simulink model "Project1_SPXMMA001"  (R2021a)
settings: Solver=ode1  StartTime=0.0  StopTime=Inf  RelTol=1e-3
InitFcn:
  |  TOFF_InitialValue.PRE = 12000;
  | OFF_InitialValue.PRE = 12000;
  | TON_InitialValue.PRE = 2000;
  | ON_InitialValue.PRE = 2000;
  | T2OFF_InitialValue.PRE = 11000;
  | T2ON_InitialValue.PRE = 3000;
  | T3OFF_InitialValue.PRE = 5000;
undefined symbols (not defined in the file): BOOL, DINT, slplc
libraries: simulink x7
(part 9 of 13)

== system Project1_SPXMMA001/PLC Controller Suite/__Logic/Task/Program/__Logic/TOF/Instruction_Enable/Initialize Function ==
  Constant : Constant  Value=0  OutDataTypeStr=BOOL
  Event Listener : EventListener  DisableCoverage=on  EventName=reset
  VarRead : Subsystem  DisableCoverage=on  TreatAsAtomicUnit=on  mask{PLCOperandTag=PRE, PLCOperandExpression=xxx_PLC_VAR_TOFF.PRE, PLCBlockType=VarRead, PLCPOUType=VarRead}
      mask prompts: PLCOperandTag "Operand Tag"
      mask init:
      | block = gcb;
      | maskObj = Simulink.Mask.get(block);
      | maskObj.Display = sprintf('disp(''%s'');', PLCOperandTag);
      | slplc.callbacks.initInstruction(gcb);
      mask Help: web([docroot '/plccoder/ref/varread' '.html']);
      mask DialogControl PLCBlockTitle Prompt: Variable Read
      mask Display: disp('PRE');
  VarWrite : Subsystem  DisableCoverage=on  TreatAsAtomicUnit=on  mask{PLCOperandTag=ACC, PLCOperandExpression=xxx_PLC_VAR_TOFF.ACC, PLCBlockType=VarWrite, PLCPOUType=VarWrite}
      mask prompts: PLCOperandTag "Operand Tag:"
      mask init:
      | slplc.callbacks.initInstruction(gcb);
      mask Help: web([docroot '/plccoder/ref/varwrite' '.html']);
      mask DialogControl PLCBlockTitle Prompt: Variable Write
      mask Display: disp(get_param(gcb, 'PLCOperandTag'));
  VarWrite1 : Subsystem  DisableCoverage=on  TreatAsAtomicUnit=on  mask{PLCOperandTag=EN, PLCOperandExpression=xxx_PLC_VAR_TOFF.EN, PLCBlockType=VarWrite, PLCPOUType=VarWrite}
      mask prompts: PLCOperandTag "Operand Tag:"
      mask init:
      | slplc.callbacks.initInstruction(gcb);
      mask Help: web([docroot '/plccoder/ref/varwrite' '.html']);
      mask DialogControl PLCBlockTitle Prompt: Variable Write
      mask Display: disp(get_param(gcb, 'PLCOperandTag'));
  VarWrite2 : Subsystem  DisableCoverage=on  TreatAsAtomicUnit=on  mask{PLCOperandTag=TT, PLCOperandExpression=xxx_PLC_VAR_TOFF.TT, PLCBlockType=VarWrite, PLCPOUType=VarWrite}
      mask prompts: PLCOperandTag "Operand Tag:"
      mask init:
      | slplc.callbacks.initInstruction(gcb);
      mask Help: web([docroot '/plccoder/ref/varwrite' '.html']);
      mask DialogControl PLCBlockTitle Prompt: Variable Write
      mask Display: disp(get_param(gcb, 'PLCOperandTag'));
  VarWrite3 : Subsystem  DisableCoverage=on  TreatAsAtomicUnit=on  mask{PLCOperandTag=DN, PLCOperandExpression=xxx_PLC_VAR_TOFF.DN, PLCBlockType=VarWrite, PLCPOUType=VarWrite}
      mask prompts: PLCOperandTag "Operand Tag:"
      mask init:
      | slplc.callbacks.initInstruction(gcb);
      mask Help: web([docroot '/plccoder/ref/varwrite' '.html']);
      mask DialogControl PLCBlockTitle Prompt: Variable Write
      mask Display: disp(get_param(gcb, 'PLCOperandTag'));
  wires:
  Constant/1 -> VarWrite1/1(In1), VarWrite2/1(In1), VarWrite3/1(In1)
  VarRead/1(Out1) -> VarWrite/1(In1)

== system Project1_SPXMMA001/PLC Controller Suite/__Logic/Task/Program/__Logic/TOF/Instruction_Enable/__CoreVarRead ==
  DataRead : DataStoreRead  DataStoreName=xxx_PLC_VAR_TOFF  IndexOptions=Index vector (dialog)  Indices=1  OutputSizes=1
  y : Outport  VectorParamsAs1DForOutWhenUnconnected=off
  wires:
  DataRead/1 -> y/1

== system Project1_SPXMMA001/PLC Controller Suite/__Logic/Task/Program/__Logic/TOF/Instruction_Enable/__CoreVarWrite ==
  u : Inport
  DataWrite : DataStoreWrite  DataStoreName=xxx_PLC_VAR_TOFF  IndexOptions=Index vector (dialog)  Indices=1  OutputSizes=1
  wires:
  u/1 -> DataWrite/1

== system Project1_SPXMMA001/PLC Controller Suite/__Logic/Task/Program/__Logic/TOF/RungInOverride/ForceRungInFalseRead ==
  __CoreLabelRead : Subsystem  Tag=CoreVarReadBlock  DisableCoverage=on  TreatAsAtomicUnit=on  mask{PLCBlockType=CoreLabelRead}
      mask init:
      | slplc.callbacks.initRoutineLabelRead(gcb);
      mask Help: web([docroot '/plccoder/ref/__corelabelread' '.html']);
      mask DialogControl PLCBlockTitle Prompt: Core Label Read
  Out1 : Outport  VectorParamsAs1DForOutWhenUnconnected=off
  wires:
  __CoreLabelRead/1(Out1) -> Out1/1

== system Project1_SPXMMA001/PLC Controller Suite/__Logic/Task/Program/__Logic/TOF1/BlockEnableRead/__CoreLabelRead ==
  DataRead : DataStoreRead  DataStoreName=x_PLCLabel__s4_3653__Block_Enable  IndexOptions=Index vector (dialog)  Indices=1  OutputSizes=1
  Out1 : Outport  VectorParamsAs1DForOutWhenUnconnected=off
  wires:
  DataRead/1 -> Out1/1

== system Project1_SPXMMA001/PLC Controller Suite/__Logic/Task/Program/__Logic/TOF1/Instruction_Enable/Initialize Function ==
  Constant : Constant  Value=0  OutDataTypeStr=BOOL
  Event Listener : EventListener  DisableCoverage=on  EventName=reset
  VarRead : Subsystem  DisableCoverage=on  TreatAsAtomicUnit=on  mask{PLCOperandTag=PRE, PLCOperandExpression=xxx_PLC_VAR_OFF.PRE, PLCBlockType=VarRead, PLCPOUType=VarRead}
      mask prompts: PLCOperandTag "Operand Tag"
      mask init:
      | block = gcb;
      | maskObj = Simulink.Mask.get(block);
      | maskObj.Display = sprintf('disp(''%s'');', PLCOperandTag);
      | slplc.callbacks.initInstruction(gcb);
      mask Help: web([docroot '/plccoder/ref/varread' '.html']);
      mask DialogControl PLCBlockTitle Prompt: Variable Read
      mask Display: disp('PRE');
  VarWrite : Subsystem  DisableCoverage=on  TreatAsAtomicUnit=on  mask{PLCOperandTag=ACC, PLCOperandExpression=xxx_PLC_VAR_OFF.ACC, PLCBlockType=VarWrite, PLCPOUType=VarWrite}
      mask prompts: PLCOperandTag "Operand Tag:"
      mask init:
      | slplc.callbacks.initInstruction(gcb);
      mask Help: web([docroot '/plccoder/ref/varwrite' '.html']);
      mask DialogControl PLCBlockTitle Prompt: Variable Write
      mask Display: disp(get_param(gcb, 'PLCOperandTag'));
  VarWrite1 : Subsystem  DisableCoverage=on  TreatAsAtomicUnit=on  mask{PLCOperandTag=EN, PLCOperandExpression=xxx_PLC_VAR_OFF.EN, PLCBlockType=VarWrite, PLCPOUType=VarWrite}
      mask prompts: PLCOperandTag "Operand Tag:"
      mask init:
      | slplc.callbacks.initInstruction(gcb);
      mask Help: web([docroot '/plccoder/ref/varwrite' '.html']);
      mask DialogControl PLCBlockTitle Prompt: Variable Write
      mask Display: disp(get_param(gcb, 'PLCOperandTag'));
  VarWrite2 : Subsystem  DisableCoverage=on  TreatAsAtomicUnit=on  mask{PLCOperandTag=TT, PLCOperandExpression=xxx_PLC_VAR_OFF.TT, PLCBlockType=VarWrite, PLCPOUType=VarWrite}
      mask prompts: PLCOperandTag "Operand Tag:"
      mask init:
      | slplc.callbacks.initInstruction(gcb);
      mask Help: web([docroot '/plccoder/ref/varwrite' '.html']);
      mask DialogControl PLCBlockTitle Prompt: Variable Write
      mask Display: disp(get_param(gcb, 'PLCOperandTag'));
  VarWrite3 : Subsystem  DisableCoverage=on  TreatAsAtomicUnit=on  mask{PLCOperandTag=DN, PLCOperandExpression=xxx_PLC_VAR_OFF.DN, PLCBlockType=VarWrite, PLCPOUType=VarWrite}
      mask prompts: PLCOperandTag "Operand Tag:"
      mask init:
      | slplc.callbacks.initInstruction(gcb);
      mask Help: web([docroot '/plccoder/ref/varwrite' '.html']);
      mask DialogControl PLCBlockTitle Prompt: Variable Write
      mask Display: disp(get_param(gcb, 'PLCOperandTag'));
  wires:
  Constant/1 -> VarWrite1/1(In1), VarWrite2/1(In1), VarWrite3/1(In1)
  VarRead/1(Out1) -> VarWrite/1(In1)

== system Project1_SPXMMA001/PLC Controller Suite/__Logic/Task/Program/__Logic/TOF1/Instruction_Enable/__CoreVarRead ==
  DataRead : DataStoreRead  DataStoreName=xxx_PLC_VAR_OFF  IndexOptions=Index vector (dialog)  Indices=1  OutputSizes=1
  y : Outport  VectorParamsAs1DForOutWhenUnconnected=off
  wires:
  DataRead/1 -> y/1

== system Project1_SPXMMA001/PLC Controller Suite/__Logic/Task/Program/__Logic/TOF1/Instruction_Enable/__CoreVarWrite ==
  u : Inport
  DataWrite : DataStoreWrite  DataStoreName=xxx_PLC_VAR_OFF  IndexOptions=Index vector (dialog)  Indices=1  OutputSizes=1
  wires:
  u/1 -> DataWrite/1

== system Project1_SPXMMA001/PLC Controller Suite/__Logic/Task/Program/__Logic/TOF1/RungInOverride/ForceRungInFalseRead ==
  __CoreLabelRead : Subsystem  Tag=CoreVarReadBlock  DisableCoverage=on  TreatAsAtomicUnit=on  mask{PLCBlockType=CoreLabelRead}
      mask init:
      | slplc.callbacks.initRoutineLabelRead(gcb);
      mask Help: web([docroot '/plccoder/ref/__corelabelread' '.html']);
      mask DialogControl PLCBlockTitle Prompt: Core Label Read
  Out1 : Outport  VectorParamsAs1DForOutWhenUnconnected=off
  wires:
  __CoreLabelRead/1(Out1) -> Out1/1

== system Project1_SPXMMA001/PLC Controller Suite/__Logic/Task/Program/__Logic/TOF2/BlockEnableRead/__CoreLabelRead ==
  DataRead : DataStoreRead  DataStoreName=x_PLCLabel__s4_3653__Block_Enable  IndexOptions=Index vector (dialog)  Indices=1  OutputSizes=1
  Out1 : Outport  VectorParamsAs1DForOutWhenUnconnected=off
  wires:
  DataRead/1 -> Out1/1

== system Project1_SPXMMA001/PLC Controller Suite/__Logic/Task/Program/__Logic/TOF2/Instruction_Enable/Initialize Function ==
  Constant : Constant  Value=0  OutDataTypeStr=BOOL
  Event Listener : EventListener  DisableCoverage=on  EventName=reset
  VarRead : Subsystem  DisableCoverage=on  TreatAsAtomicUnit=on  mask{PLCOperandTag=PRE, PLCOperandExpression=xxx_PLC_VAR_T2OFF.PRE, PLCBlockType=VarRead, PLCPOUType=VarRead}
      mask prompts: PLCOperandTag "Operand Tag"
      mask init:
      | block = gcb;
      | maskObj = Simulink.Mask.get(block);
      | maskObj.Display = sprintf('disp(''%s'');', PLCOperandTag);
      | slplc.callbacks.initInstruction(gcb);
      mask Help: web([docroot '/plccoder/ref/varread' '.html']);
      mask DialogControl PLCBlockTitle Prompt: Variable Read
      mask Display: disp('PRE');
  VarWrite : Subsystem  DisableCoverage=on  TreatAsAtomicUnit=on  mask{PLCOperandTag=ACC, PLCOperandExpression=xxx_PLC_VAR_T2OFF.ACC, PLCBlockType=VarWrite, PLCPOUType=VarWrite}
      mask prompts: PLCOperandTag "Operand Tag:"
      mask init:
      | slplc.callbacks.initInstruction(gcb);
      mask Help: web([docroot '/plccoder/ref/varwrite' '.html']);
      mask DialogControl PLCBlockTitle Prompt: Variable Write
      mask Display: disp(get_param(gcb, 'PLCOperandTag'));
  VarWrite1 : Subsystem  DisableCoverage=on  TreatAsAtomicUnit=on  mask{PLCOperandTag=EN, PLCOperandExpression=xxx_PLC_VAR_T2OFF.EN, PLCBlockType=VarWrite, PLCPOUType=VarWrite}
      mask prompts: PLCOperandTag "Operand Tag:"
      mask init:
      | slplc.callbacks.initInstruction(gcb);
      mask Help: web([docroot '/plccoder/ref/varwrite' '.html']);
      mask DialogControl PLCBlockTitle Prompt: Variable Write
      mask Display: disp(get_param(gcb, 'PLCOperandTag'));
  VarWrite2 : Subsystem  DisableCoverage=on  TreatAsAtomicUnit=on  mask{PLCOperandTag=TT, PLCOperandExpression=xxx_PLC_VAR_T2OFF.TT, PLCBlockType=VarWrite, PLCPOUType=VarWrite}
      mask prompts: PLCOperandTag "Operand Tag:"
      mask init:
      | slplc.callbacks.initInstruction(gcb);
      mask Help: web([docroot '/plccoder/ref/varwrite' '.html']);
      mask DialogControl PLCBlockTitle Prompt: Variable Write
      mask Display: disp(get_param(gcb, 'PLCOperandTag'));
  VarWrite3 : Subsystem  DisableCoverage=on  TreatAsAtomicUnit=on  mask{PLCOperandTag=DN, PLCOperandExpression=xxx_PLC_VAR_T2OFF.DN, PLCBlockType=VarWrite, PLCPOUType=VarWrite}
      mask prompts: PLCOperandTag "Operand Tag:"
      mask init:
      | slplc.callbacks.initInstruction(gcb);
      mask Help: web([docroot '/plccoder/ref/varwrite' '.html']);
      mask DialogControl PLCBlockTitle Prompt: Variable Write
      mask Display: disp(get_param(gcb, 'PLCOperandTag'));
  wires:
  Constant/1 -> VarWrite1/1(In1), VarWrite2/1(In1), VarWrite3/1(In1)
  VarRead/1(Out1) -> VarWrite/1(In1)

== system Project1_SPXMMA001/PLC Controller Suite/__Logic/Task/Program/__Logic/TOF2/Instruction_Enable/__CoreVarRead ==
  DataRead : DataStoreRead  DataStoreName=xxx_PLC_VAR_T2OFF  IndexOptions=Index vector (dialog)  Indices=1  OutputSizes=1
  y : Outport  VectorParamsAs1DForOutWhenUnconnected=off
  wires:
  DataRead/1 -> y/1

== system Project1_SPXMMA001/PLC Controller Suite/__Logic/Task/Program/__Logic/TOF2/Instruction_Enable/__CoreVarWrite ==
  u : Inport
  DataWrite : DataStoreWrite  DataStoreName=xxx_PLC_VAR_T2OFF  IndexOptions=Index vector (dialog)  Indices=1  OutputSizes=1
  wires:
  u/1 -> DataWrite/1

== system Project1_SPXMMA001/PLC Controller Suite/__Logic/Task/Program/__Logic/TOF2/RungInOverride/ForceRungInFalseRead ==
  __CoreLabelRead : Subsystem  Tag=CoreVarReadBlock  DisableCoverage=on  TreatAsAtomicUnit=on  mask{PLCBlockType=CoreLabelRead}
      mask init:
      | slplc.callbacks.initRoutineLabelRead(gcb);
      mask Help: web([docroot '/plccoder/ref/__corelabelread' '.html']);
      mask DialogControl PLCBlockTitle Prompt: Core Label Read
  Out1 : Outport  VectorParamsAs1DForOutWhenUnconnected=off
  wires:
  __CoreLabelRead/1(Out1) -> Out1/1

== system Project1_SPXMMA001/PLC Controller Suite/__Logic/Task/Program/__Logic/TOF3/BlockEnableRead/__CoreLabelRead ==
  DataRead : DataStoreRead  DataStoreName=x_PLCLabel__s4_3653__Block_Enable  IndexOptions=Index vector (dialog)  Indices=1  OutputSizes=1
  Out1 : Outport  VectorParamsAs1DForOutWhenUnconnected=off
  wires:
  DataRead/1 -> Out1/1

== system Project1_SPXMMA001/PLC Controller Suite/__Logic/Task/Program/__Logic/TOF3/Instruction_Enable/Initialize Function ==
  Constant : Constant  Value=0  OutDataTypeStr=BOOL
  Event Listener : EventListener  DisableCoverage=on  EventName=reset
  VarRead : Subsystem  DisableCoverage=on  TreatAsAtomicUnit=on  mask{PLCOperandTag=PRE, PLCOperandExpression=xxx_PLC_VAR_T3OFF.PRE, PLCBlockType=VarRead, PLCPOUType=VarRead}
      mask prompts: PLCOperandTag "Operand Tag"
      mask init:
      | block = gcb;
      | maskObj = Simulink.Mask.get(block);
      | maskObj.Display = sprintf('disp(''%s'');', PLCOperandTag);
      | slplc.callbacks.initInstruction(gcb);
      mask Help: web([docroot '/plccoder/ref/varread' '.html']);
      mask DialogControl PLCBlockTitle Prompt: Variable Read
      mask Display: disp('PRE');
  VarWrite : Subsystem  DisableCoverage=on  TreatAsAtomicUnit=on  mask{PLCOperandTag=ACC, PLCOperandExpression=xxx_PLC_VAR_T3OFF.ACC, PLCBlockType=VarWrite, PLCPOUType=VarWrite}
      mask prompts: PLCOperandTag "Operand Tag:"
      mask init:
      | slplc.callbacks.initInstruction(gcb);
      mask Help: web([docroot '/plccoder/ref/varwrite' '.html']);
      mask DialogControl PLCBlockTitle Prompt: Variable Write
      mask Display: disp(get_param(gcb, 'PLCOperandTag'));
  VarWrite1 : Subsystem  DisableCoverage=on  TreatAsAtomicUnit=on  mask{PLCOperandTag=EN, PLCOperandExpression=xxx_PLC_VAR_T3OFF.EN, PLCBlockType=VarWrite, PLCPOUType=VarWrite}
      mask prompts: PLCOperandTag "Operand Tag:"
      mask init:
      | slplc.callbacks.initInstruction(gcb);
      mask Help: web([docroot '/plccoder/ref/varwrite' '.html']);
      mask DialogControl PLCBlockTitle Prompt: Variable Write
      mask Display: disp(get_param(gcb, 'PLCOperandTag'));
  VarWrite2 : Subsystem  DisableCoverage=on  TreatAsAtomicUnit=on  mask{PLCOperandTag=TT, PLCOperandExpression=xxx_PLC_VAR_T3OFF.TT, PLCBlockType=VarWrite, PLCPOUType=VarWrite}
      mask prompts: PLCOperandTag "Operand Tag:"
      mask init:
      | slplc.callbacks.initInstruction(gcb);
      mask Help: web([docroot '/plccoder/ref/varwrite' '.html']);
      mask DialogControl PLCBlockTitle Prompt: Variable Write
      mask Display: disp(get_param(gcb, 'PLCOperandTag'));
  VarWrite3 : Subsystem  DisableCoverage=on  TreatAsAtomicUnit=on  mask{PLCOperandTag=DN, PLCOperandExpression=xxx_PLC_VAR_T3OFF.DN, PLCBlockType=VarWrite, PLCPOUType=VarWrite}
      mask prompts: PLCOperandTag "Operand Tag:"
      mask init:
      | slplc.callbacks.initInstruction(gcb);
      mask Help: web([docroot '/plccoder/ref/varwrite' '.html']);
      mask DialogControl PLCBlockTitle Prompt: Variable Write
      mask Display: disp(get_param(gcb, 'PLCOperandTag'));
  wires:
  Constant/1 -> VarWrite1/1(In1), VarWrite2/1(In1), VarWrite3/1(In1)
  VarRead/1(Out1) -> VarWrite/1(In1)

== system Project1_SPXMMA001/PLC Controller Suite/__Logic/Task/Program/__Logic/TOF3/Instruction_Enable/__CoreVarRead ==
  DataRead : DataStoreRead  DataStoreName=xxx_PLC_VAR_T3OFF  IndexOptions=Index vector (dialog)  Indices=1  OutputSizes=1
  y : Outport  VectorParamsAs1DForOutWhenUnconnected=off
  wires:
  DataRead/1 -> y/1

== system Project1_SPXMMA001/PLC Controller Suite/__Logic/Task/Program/__Logic/TOF3/Instruction_Enable/__CoreVarWrite ==
  u : Inport
  DataWrite : DataStoreWrite  DataStoreName=xxx_PLC_VAR_T3OFF  IndexOptions=Index vector (dialog)  Indices=1  OutputSizes=1
  wires:
  u/1 -> DataWrite/1

== system Project1_SPXMMA001/PLC Controller Suite/__Logic/Task/Program/__Logic/TOF3/RungInOverride/ForceRungInFalseRead ==
  __CoreLabelRead : Subsystem  Tag=CoreVarReadBlock  DisableCoverage=on  TreatAsAtomicUnit=on  mask{PLCBlockType=CoreLabelRead}
      mask init:
      | slplc.callbacks.initRoutineLabelRead(gcb);
      mask Help: web([docroot '/plccoder/ref/__corelabelread' '.html']);
      mask DialogControl PLCBlockTitle Prompt: Core Label Read
  Out1 : Outport  VectorParamsAs1DForOutWhenUnconnected=off
  wires:
  __CoreLabelRead/1(Out1) -> Out1/1

== system Project1_SPXMMA001/PLC Controller Suite/__Logic/Task/Program/__Logic/TON/BlockEnableRead/__CoreLabelRead ==
  DataRead : DataStoreRead  DataStoreName=x_PLCLabel__s4_3653__Block_Enable  IndexOptions=Index vector (dialog)  Indices=1  OutputSizes=1
  Out1 : Outport  VectorParamsAs1DForOutWhenUnconnected=off
  wires:
  DataRead/1 -> Out1/1

== system Project1_SPXMMA001/PLC Controller Suite/__Logic/Task/Program/__Logic/TON/Instruction_Enable/Initialize Function ==
  Constant : Constant  Value=0  OutDataTypeStr=BOOL
  Constant1 : Constant  Value=0  OutDataTypeStr=DINT
  Event Listener : EventListener  DisableCoverage=on  EventName=reset
  VarWrite : Subsystem  DisableCoverage=on  TreatAsAtomicUnit=on  mask{PLCOperandTag=ACC, PLCOperandExpression=xxx_PLC_VAR_TON.ACC, PLCBlockType=VarWrite, PLCPOUType=VarWrite}
      mask prompts: PLCOperandTag "Operand Tag:"
      mask init:
      | slplc.callbacks.initInstruction(gcb);
      mask Help: web([docroot '/plccoder/ref/varwrite' '.html']);
      mask DialogControl PLCBlockTitle Prompt: Variable Write
      mask Display: disp(get_param(gcb, 'PLCOperandTag'));
  VarWrite1 : Subsystem  DisableCoverage=on  TreatAsAtomicUnit=on  mask{PLCOperandTag=EN, PLCOperandExpression=xxx_PLC_VAR_TON.EN, PLCBlockType=VarWrite, PLCPOUType=VarWrite}
      mask prompts: PLCOperandTag "Operand Tag:"
      mask init:
      | slplc.callbacks.initInstruction(gcb);
      mask Help: web([docroot '/plccoder/ref/varwrite' '.html']);
      mask DialogControl PLCBlockTitle Prompt: Variable Write
      mask Display: disp(get_param(gcb, 'PLCOperandTag'));
  VarWrite2 : Subsystem  DisableCoverage=on  TreatAsAtomicUnit=on  mask{PLCOperandTag=TT, PLCOperandExpression=xxx_PLC_VAR_TON.TT, PLCBlockType=VarWrite, PLCPOUType=VarWrite}
      mask prompts: PLCOperandTag "Operand Tag:"
      mask init:
      | slplc.callbacks.initInstruction(gcb);
      mask Help: web([docroot '/plccoder/ref/varwrite' '.html']);
      mask DialogControl PLCBlockTitle Prompt: Variable Write
      mask Display: disp(get_param(gcb, 'PLCOperandTag'));
  VarWrite3 : Subsystem  DisableCoverage=on  TreatAsAtomicUnit=on  mask{PLCOperandTag=DN, PLCOperandExpression=xxx_PLC_VAR_TON.DN, PLCBlockType=VarWrite, PLCPOUType=VarWrite}
      mask prompts: PLCOperandTag "Operand Tag:"
      mask init:
      | slplc.callbacks.initInstruction(gcb);
      mask Help: web([docroot '/plccoder/ref/varwrite' '.html']);
      mask DialogControl PLCBlockTitle Prompt: Variable Write
      mask Display: disp(get_param(gcb, 'PLCOperandTag'));
  wires:
  Constant/1 -> VarWrite1/1(In1), VarWrite2/1(In1), VarWrite3/1(In1)
  Constant1/1 -> VarWrite/1(In1)

== system Project1_SPXMMA001/PLC Controller Suite/__Logic/Task/Program/__Logic/TON/Instruction_Enable/__CoreVarRead ==
  DataRead : DataStoreRead  DataStoreName=xxx_PLC_VAR_TON  IndexOptions=Index vector (dialog)  Indices=1  OutputSizes=1
  y : Outport  VectorParamsAs1DForOutWhenUnconnected=off
  wires:
  DataRead/1 -> y/1

== system Project1_SPXMMA001/PLC Controller Suite/__Logic/Task/Program/__Logic/TON/Instruction_Enable/__CoreVarWrite ==
  u : Inport
  DataWrite : DataStoreWrite  DataStoreName=xxx_PLC_VAR_TON  IndexOptions=Index vector (dialog)  Indices=1  OutputSizes=1
  wires:
  u/1 -> DataWrite/1

== system Project1_SPXMMA001/PLC Controller Suite/__Logic/Task/Program/__Logic/TON/RungInOverride/ForceRungInFalseRead ==
  __CoreLabelRead : Subsystem  Tag=CoreVarReadBlock  DisableCoverage=on  TreatAsAtomicUnit=on  mask{PLCBlockType=CoreLabelRead}
      mask init:
      | slplc.callbacks.initRoutineLabelRead(gcb);
      mask Help: web([docroot '/plccoder/ref/__corelabelread' '.html']);
      mask DialogControl PLCBlockTitle Prompt: Core Label Read
  Out1 : Outport  VectorParamsAs1DForOutWhenUnconnected=off
  wires:
  __CoreLabelRead/1(Out1) -> Out1/1

== system Project1_SPXMMA001/PLC Controller Suite/__Logic/Task/Program/__Logic/TON1/BlockEnableRead/__CoreLabelRead ==
  DataRead : DataStoreRead  DataStoreName=x_PLCLabel__s4_3653__Block_Enable  IndexOptions=Index vector (dialog)  Indices=1  OutputSizes=1
  Out1 : Outport  VectorParamsAs1DForOutWhenUnconnected=off
  wires:
  DataRead/1 -> Out1/1

== system Project1_SPXMMA001/PLC Controller Suite/__Logic/Task/Program/__Logic/TON1/Instruction_Enable/Initialize Function ==
  Constant : Constant  Value=0  OutDataTypeStr=BOOL
  Constant1 : Constant  Value=0  OutDataTypeStr=DINT
  Event Listener : EventListener  DisableCoverage=on  EventName=reset
  VarWrite : Subsystem  DisableCoverage=on  TreatAsAtomicUnit=on  mask{PLCOperandTag=ACC, PLCOperandExpression=xxx_PLC_VAR_ON.ACC, PLCBlockType=VarWrite, PLCPOUType=VarWrite}
      mask prompts: PLCOperandTag "Operand Tag:"
      mask init:
      | slplc.callbacks.initInstruction(gcb);
      mask Help: web([docroot '/plccoder/ref/varwrite' '.html']);
      mask DialogControl PLCBlockTitle Prompt: Variable Write
      mask Display: disp(get_param(gcb, 'PLCOperandTag'));
  VarWrite1 : Subsystem  DisableCoverage=on  TreatAsAtomicUnit=on  mask{PLCOperandTag=EN, PLCOperandExpression=xxx_PLC_VAR_ON.EN, PLCBlockType=VarWrite, PLCPOUType=VarWrite}
      mask prompts: PLCOperandTag "Operand Tag:"
      mask init:
      | slplc.callbacks.initInstruction(gcb);
      mask Help: web([docroot '/plccoder/ref/varwrite' '.html']);
      mask DialogControl PLCBlockTitle Prompt: Variable Write
      mask Display: disp(get_param(gcb, 'PLCOperandTag'));
  VarWrite2 : Subsystem  DisableCoverage=on  TreatAsAtomicUnit=on  mask{PLCOperandTag=TT, PLCOperandExpression=xxx_PLC_VAR_ON.TT, PLCBlockType=VarWrite, PLCPOUType=VarWrite}
      mask prompts: PLCOperandTag "Operand Tag:"
      mask init:
      | slplc.callbacks.initInstruction(gcb);
      mask Help: web([docroot '/plccoder/ref/varwrite' '.html']);
      mask DialogControl PLCBlockTitle Prompt: Variable Write
      mask Display: disp(get_param(gcb, 'PLCOperandTag'));
  VarWrite3 : Subsystem  DisableCoverage=on  TreatAsAtomicUnit=on  mask{PLCOperandTag=DN, PLCOperandExpression=xxx_PLC_VAR_ON.DN, PLCBlockType=VarWrite, PLCPOUType=VarWrite}
      mask prompts: PLCOperandTag "Operand Tag:"
      mask init:
      | slplc.callbacks.initInstruction(gcb);
      mask Help: web([docroot '/plccoder/ref/varwrite' '.html']);
      mask DialogControl PLCBlockTitle Prompt: Variable Write
      mask Display: disp(get_param(gcb, 'PLCOperandTag'));
  wires:
  Constant/1 -> VarWrite1/1(In1), VarWrite2/1(In1), VarWrite3/1(In1)
  Constant1/1 -> VarWrite/1(In1)

== system Project1_SPXMMA001/PLC Controller Suite/__Logic/Task/Program/__Logic/TON1/Instruction_Enable/__CoreVarRead ==
  DataRead : DataStoreRead  DataStoreName=xxx_PLC_VAR_ON  IndexOptions=Index vector (dialog)  Indices=1  OutputSizes=1
  y : Outport  VectorParamsAs1DForOutWhenUnconnected=off
  wires:
  DataRead/1 -> y/1

== system Project1_SPXMMA001/PLC Controller Suite/__Logic/Task/Program/__Logic/TON1/Instruction_Enable/__CoreVarWrite ==
  u : Inport
  DataWrite : DataStoreWrite  DataStoreName=xxx_PLC_VAR_ON  IndexOptions=Index vector (dialog)  Indices=1  OutputSizes=1
  wires:
  u/1 -> DataWrite/1

== system Project1_SPXMMA001/PLC Controller Suite/__Logic/Task/Program/__Logic/TON1/RungInOverride/ForceRungInFalseRead ==
  __CoreLabelRead : Subsystem  Tag=CoreVarReadBlock  DisableCoverage=on  TreatAsAtomicUnit=on  mask{PLCBlockType=CoreLabelRead}
      mask init:
      | slplc.callbacks.initRoutineLabelRead(gcb);
      mask Help: web([docroot '/plccoder/ref/__corelabelread' '.html']);
      mask DialogControl PLCBlockTitle Prompt: Core Label Read
  Out1 : Outport  VectorParamsAs1DForOutWhenUnconnected=off
  wires:
  __CoreLabelRead/1(Out1) -> Out1/1

== system Project1_SPXMMA001/PLC Controller Suite/__Logic/Task/Program/__Logic/TON2/BlockEnableRead/__CoreLabelRead ==
  DataRead : DataStoreRead  DataStoreName=x_PLCLabel__s4_3653__Block_Enable  IndexOptions=Index vector (dialog)  Indices=1  OutputSizes=1
  Out1 : Outport  VectorParamsAs1DForOutWhenUnconnected=off
  wires:
  DataRead/1 -> Out1/1

== system Project1_SPXMMA001/PLC Controller Suite/__Logic/Task/Program/__Logic/TON2/Instruction_Enable/Initialize Function ==
  Constant : Constant  Value=0  OutDataTypeStr=BOOL
  Constant1 : Constant  Value=0  OutDataTypeStr=DINT
  Event Listener : EventListener  DisableCoverage=on  EventName=reset
  VarWrite : Subsystem  DisableCoverage=on  TreatAsAtomicUnit=on  mask{PLCOperandTag=ACC, PLCOperandExpression=xxx_PLC_VAR_T2ON.ACC, PLCBlockType=VarWrite, PLCPOUType=VarWrite}
      mask prompts: PLCOperandTag "Operand Tag:"
      mask init:
      | slplc.callbacks.initInstruction(gcb);
      mask Help: web([docroot '/plccoder/ref/varwrite' '.html']);
      mask DialogControl PLCBlockTitle Prompt: Variable Write
      mask Display: disp(get_param(gcb, 'PLCOperandTag'));
  VarWrite1 : Subsystem  DisableCoverage=on  TreatAsAtomicUnit=on  mask{PLCOperandTag=EN, PLCOperandExpression=xxx_PLC_VAR_T2ON.EN, PLCBlockType=VarWrite, PLCPOUType=VarWrite}
      mask prompts: PLCOperandTag "Operand Tag:"
      mask init:
      | slplc.callbacks.initInstruction(gcb);
      mask Help: web([docroot '/plccoder/ref/varwrite' '.html']);
      mask DialogControl PLCBlockTitle Prompt: Variable Write
      mask Display: disp(get_param(gcb, 'PLCOperandTag'));
  VarWrite2 : Subsystem  DisableCoverage=on  TreatAsAtomicUnit=on  mask{PLCOperandTag=TT, PLCOperandExpression=xxx_PLC_VAR_T2ON.TT, PLCBlockType=VarWrite, PLCPOUType=VarWrite}
      mask prompts: PLCOperandTag "Operand Tag:"
      mask init:
      | slplc.callbacks.initInstruction(gcb);
      mask Help: web([docroot '/plccoder/ref/varwrite' '.html']);
      mask DialogControl PLCBlockTitle Prompt: Variable Write
      mask Display: disp(get_param(gcb, 'PLCOperandTag'));
  VarWrite3 : Subsystem  DisableCoverage=on  TreatAsAtomicUnit=on  mask{PLCOperandTag=DN, PLCOperandExpression=xxx_PLC_VAR_T2ON.DN, PLCBlockType=VarWrite, PLCPOUType=VarWrite}
      mask prompts: PLCOperandTag "Operand Tag:"
      mask init:
      | slplc.callbacks.initInstruction(gcb);
      mask Help: web([docroot '/plccoder/ref/varwrite' '.html']);
      mask DialogControl PLCBlockTitle Prompt: Variable Write
      mask Display: disp(get_param(gcb, 'PLCOperandTag'));
  wires:
  Constant/1 -> VarWrite1/1(In1), VarWrite2/1(In1), VarWrite3/1(In1)
  Constant1/1 -> VarWrite/1(In1)

== system Project1_SPXMMA001/PLC Controller Suite/__Logic/Task/Program/__Logic/TON2/Instruction_Enable/__CoreVarRead ==
  DataRead : DataStoreRead  DataStoreName=xxx_PLC_VAR_T2ON  IndexOptions=Index vector (dialog)  Indices=1  OutputSizes=1
  y : Outport  VectorParamsAs1DForOutWhenUnconnected=off
  wires:
  DataRead/1 -> y/1

== system Project1_SPXMMA001/PLC Controller Suite/__Logic/Task/Program/__Logic/TON2/Instruction_Enable/__CoreVarWrite ==
  u : Inport
  DataWrite : DataStoreWrite  DataStoreName=xxx_PLC_VAR_T2ON  IndexOptions=Index vector (dialog)  Indices=1  OutputSizes=1
  wires:
  u/1 -> DataWrite/1

== system Project1_SPXMMA001/PLC Controller Suite/__Logic/Task/Program/__Logic/TON2/RungInOverride/ForceRungInFalseRead ==
  __CoreLabelRead : Subsystem  Tag=CoreVarReadBlock  DisableCoverage=on  TreatAsAtomicUnit=on  mask{PLCBlockType=CoreLabelRead}
      mask init:
      | slplc.callbacks.initRoutineLabelRead(gcb);
      mask Help: web([docroot '/plccoder/ref/__corelabelread' '.html']);
      mask DialogControl PLCBlockTitle Prompt: Core Label Read
  Out1 : Outport  VectorParamsAs1DForOutWhenUnconnected=off
  wires:
  __CoreLabelRead/1(Out1) -> Out1/1

== system Project1_SPXMMA001/PLC Controller Suite/__Logic/Task/Program/__Logic/XIC/BlockEnableRead/__CoreLabelRead ==
  DataRead : DataStoreRead  DataStoreName=x_PLCLabel__s4_3653__Block_Enable  IndexOptions=Index vector (dialog)  Indices=1  OutputSizes=1
  Out1 : Outport  VectorParamsAs1DForOutWhenUnconnected=off
  wires:
  DataRead/1 -> Out1/1

== system Project1_SPXMMA001/PLC Controller Suite/__Logic/Task/Program/__Logic/XIC/Instruction_Enable/__CoreVarRead ==
  DataRead : DataStoreRead  DataStoreName=xxx_PLC_VAR_PED1_1  IndexOptions=Index vector (dialog)  Indices=1  OutputSizes=1
  y : Outport  VectorParamsAs1DForOutWhenUnconnected=off
  wires:
  DataRead/1 -> y/1

== system Project1_SPXMMA001/PLC Controller Suite/__Logic/Task/Program/__Logic/XIC/RungInOverride/ForceRungInFalseRead ==
  __CoreLabelRead : Subsystem  Tag=CoreVarReadBlock  DisableCoverage=on  TreatAsAtomicUnit=on  mask{PLCBlockType=CoreLabelRead}
      mask init:
      | slplc.callbacks.initRoutineLabelRead(gcb);
      mask Help: web([docroot '/plccoder/ref/__corelabelread' '.html']);
      mask DialogControl PLCBlockTitle Prompt: Core Label Read
  Out1 : Outport  VectorParamsAs1DForOutWhenUnconnected=off
  wires:
  __CoreLabelRead/1(Out1) -> Out1/1

== system Project1_SPXMMA001/PLC Controller Suite/__Logic/Task/Program/__Logic/XIC1/BlockEnableRead/__CoreLabelRead ==
  DataRead : DataStoreRead  DataStoreName=x_PLCLabel__s4_3653__Block_Enable  IndexOptions=Index vector (dialog)  Indices=1  OutputSizes=1
  Out1 : Outport  VectorParamsAs1DForOutWhenUnconnected=off
  wires:
  DataRead/1 -> Out1/1

== system Project1_SPXMMA001/PLC Controller Suite/__Logic/Task/Program/__Logic/XIC1/Instruction_Enable/__CoreVarRead ==
  DataRead : DataStoreRead  DataStoreName=xxx_PLC_VAR_PED1_2  IndexOptions=Index vector (dialog)  Indices=1  OutputSizes=1
  y : Outport  VectorParamsAs1DForOutWhenUnconnected=off
  wires:
  DataRead/1 -> y/1

== system Project1_SPXMMA001/PLC Controller Suite/__Logic/Task/Program/__Logic/XIC1/RungInOverride/ForceRungInFalseRead ==
  __CoreLabelRead : Subsystem  Tag=CoreVarReadBlock  DisableCoverage=on  TreatAsAtomicUnit=on  mask{PLCBlockType=CoreLabelRead}
      mask init:
      | slplc.callbacks.initRoutineLabelRead(gcb);
      mask Help: web([docroot '/plccoder/ref/__corelabelread' '.html']);
      mask DialogControl PLCBlockTitle Prompt: Core Label Read
  Out1 : Outport  VectorParamsAs1DForOutWhenUnconnected=off
  wires:
  __CoreLabelRead/1(Out1) -> Out1/1

== system Project1_SPXMMA001/PLC Controller Suite/__Logic/Task/Program/__Logic/XIC10/BlockEnableRead/__CoreLabelRead ==
  DataRead : DataStoreRead  DataStoreName=x_PLCLabel__s4_3653__Block_Enable  IndexOptions=Index vector (dialog)  Indices=1  OutputSizes=1
  Out1 : Outport  VectorParamsAs1DForOutWhenUnconnected=off
  wires:
  DataRead/1 -> Out1/1

== system Project1_SPXMMA001/PLC Controller Suite/__Logic/Task/Program/__Logic/XIC10/Instruction_Enable/__CoreVarRead ==
  DataRead : DataStoreRead  DataStoreName=xxx_PLC_VAR_T2ON  DataStoreElements=xxx_PLC_VAR_T2ON.DN  IndexOptions=Index vector (dialog)  Indices=1  OutputSizes=1
  y : Outport  VectorParamsAs1DForOutWhenUnconnected=off
  wires:
  DataRead/1 -> y/1

== system Project1_SPXMMA001/PLC Controller Suite/__Logic/Task/Program/__Logic/XIC10/RungInOverride/ForceRungInFalseRead ==
  __CoreLabelRead : Subsystem  Tag=CoreVarReadBlock  DisableCoverage=on  TreatAsAtomicUnit=on  mask{PLCBlockType=CoreLabelRead}
      mask init:
      | slplc.callbacks.initRoutineLabelRead(gcb);
      mask Help: web([docroot '/plccoder/ref/__corelabelread' '.html']);
      mask DialogControl PLCBlockTitle Prompt: Core Label Read
  Out1 : Outport  VectorParamsAs1DForOutWhenUnconnected=off
  wires:
  __CoreLabelRead/1(Out1) -> Out1/1

== system Project1_SPXMMA001/PLC Controller Suite/__Logic/Task/Program/__Logic/XIC11/BlockEnableRead/__CoreLabelRead ==
  DataRead : DataStoreRead  DataStoreName=x_PLCLabel__s4_3653__Block_Enable  IndexOptions=Index vector (dialog)  Indices=1  OutputSizes=1
  Out1 : Outport  VectorParamsAs1DForOutWhenUnconnected=off
  wires:
  DataRead/1 -> Out1/1

== system Project1_SPXMMA001/PLC Controller Suite/__Logic/Task/Program/__Logic/XIC11/Instruction_Enable/__CoreVarRead ==
  DataRead : DataStoreRead  DataStoreName=xxx_PLC_VAR_ZONE1_SENSOR  IndexOptions=Index vector (dialog)  Indices=1  OutputSizes=1
  y : Outport  VectorParamsAs1DForOutWhenUnconnected=off
  wires:
  DataRead/1 -> y/1

== system Project1_SPXMMA001/PLC Controller Suite/__Logic/Task/Program/__Logic/XIC11/RungInOverride/ForceRungInFalseRead ==
  __CoreLabelRead : Subsystem  Tag=CoreVarReadBlock  DisableCoverage=on  TreatAsAtomicUnit=on  mask{PLCBlockType=CoreLabelRead}
      mask init:
      | slplc.callbacks.initRoutineLabelRead(gcb);
      mask Help: web([docroot '/plccoder/ref/__corelabelread' '.html']);
      mask DialogControl PLCBlockTitle Prompt: Core Label Read
  Out1 : Outport  VectorParamsAs1DForOutWhenUnconnected=off
  wires:
  __CoreLabelRead/1(Out1) -> Out1/1

== system Project1_SPXMMA001/PLC Controller Suite/__Logic/Task/Program/__Logic/XIC12/BlockEnableRead/__CoreLabelRead ==
  DataRead : DataStoreRead  DataStoreName=x_PLCLabel__s4_3653__Block_Enable  IndexOptions=Index vector (dialog)  Indices=1  OutputSizes=1
  Out1 : Outport  VectorParamsAs1DForOutWhenUnconnected=off
  wires:
  DataRead/1 -> Out1/1

== system Project1_SPXMMA001/PLC Controller Suite/__Logic/Task/Program/__Logic/XIC12/Instruction_Enable/__CoreVarRead ==
  DataRead : DataStoreRead  DataStoreName=xxx_PLC_VAR_ZONE1_SENSOR  IndexOptions=Index vector (dialog)  Indices=1  OutputSizes=1
  y : Outport  VectorParamsAs1DForOutWhenUnconnected=off
  wires:
  DataRead/1 -> y/1

== system Project1_SPXMMA001/PLC Controller Suite/__Logic/Task/Program/__Logic/XIC12/RungInOverride/ForceRungInFalseRead ==
  __CoreLabelRead : Subsystem  Tag=CoreVarReadBlock  DisableCoverage=on  TreatAsAtomicUnit=on  mask{PLCBlockType=CoreLabelRead}
      mask init:
      | slplc.callbacks.initRoutineLabelRead(gcb);
      mask Help: web([docroot '/plccoder/ref/__corelabelread' '.html']);
      mask DialogControl PLCBlockTitle Prompt: Core Label Read
  Out1 : Outport  VectorParamsAs1DForOutWhenUnconnected=off
  wires:
  __CoreLabelRead/1(Out1) -> Out1/1

== system Project1_SPXMMA001/PLC Controller Suite/__Logic/Task/Program/__Logic/XIC13/BlockEnableRead/__CoreLabelRead ==
  DataRead : DataStoreRead  DataStoreName=x_PLCLabel__s4_3653__Block_Enable  IndexOptions=Index vector (dialog)  Indices=1  OutputSizes=1
  Out1 : Outport  VectorParamsAs1DForOutWhenUnconnected=off
  wires:
  DataRead/1 -> Out1/1

== system Project1_SPXMMA001/PLC Controller Suite/__Logic/Task/Program/__Logic/XIC13/Instruction_Enable/__CoreVarRead ==
  DataRead : DataStoreRead  DataStoreName=xxx_PLC_VAR_ZONE2  IndexOptions=Index vector (dialog)  Indices=1  OutputSizes=1
  y : Outport  VectorParamsAs1DForOutWhenUnconnected=off
  wires:
  DataRead/1 -> y/1

== system Project1_SPXMMA001/PLC Controller Suite/__Logic/Task/Program/__Logic/XIC13/RungInOverride/ForceRungInFalseRead ==
  __CoreLabelRead : Subsystem  Tag=CoreVarReadBlock  DisableCoverage=on  TreatAsAtomicUnit=on  mask{PLCBlockType=CoreLabelRead}
      mask init:
      | slplc.callbacks.initRoutineLabelRead(gcb);
      mask Help: web([docroot '/plccoder/ref/__corelabelread' '.html']);
      mask DialogControl PLCBlockTitle Prompt: Core Label Read
  Out1 : Outport  VectorParamsAs1DForOutWhenUnconnected=off
  wires:
  __CoreLabelRead/1(Out1) -> Out1/1

== system Project1_SPXMMA001/PLC Controller Suite/__Logic/Task/Program/__Logic/XIC14/BlockEnableRead/__CoreLabelRead ==
  DataRead : DataStoreRead  DataStoreName=x_PLCLabel__s4_3653__Block_Enable  IndexOptions=Index vector (dialog)  Indices=1  OutputSizes=1
  Out1 : Outport  VectorParamsAs1DForOutWhenUnconnected=off
  wires:
  DataRead/1 -> Out1/1

== system Project1_SPXMMA001/PLC Controller Suite/__Logic/Task/Program/__Logic/XIC14/Instruction_Enable/__CoreVarRead ==
  DataRead : DataStoreRead  DataStoreName=xxx_PLC_VAR_T3OFF  DataStoreElements=xxx_PLC_VAR_T3OFF.DN  IndexOptions=Index vector (dialog)  Indices=1  OutputSizes=1
  y : Outport  VectorParamsAs1DForOutWhenUnconnected=off
  wires:
  DataRead/1 -> y/1

== system Project1_SPXMMA001/PLC Controller Suite/__Logic/Task/Program/__Logic/XIC14/RungInOverride/ForceRungInFalseRead ==
  __CoreLabelRead : Subsystem  Tag=CoreVarReadBlock  DisableCoverage=on  TreatAsAtomicUnit=on  mask{PLCBlockType=CoreLabelRead}
      mask init:
      | slplc.callbacks.initRoutineLabelRead(gcb);
      mask Help: web([docroot '/plccoder/ref/__corelabelread' '.html']);
      mask DialogControl PLCBlockTitle Prompt: Core Label Read
  Out1 : Outport  VectorParamsAs1DForOutWhenUnconnected=off
  wires:
  __CoreLabelRead/1(Out1) -> Out1/1

== system Project1_SPXMMA001/PLC Controller Suite/__Logic/Task/Program/__Logic/XIC16/BlockEnableRead/__CoreLabelRead ==
  DataRead : DataStoreRead  DataStoreName=x_PLCLabel__s4_3653__Block_Enable  IndexOptions=Index vector (dialog)  Indices=1  OutputSizes=1
  Out1 : Outport  VectorParamsAs1DForOutWhenUnconnected=off
  wires:
  DataRead/1 -> Out1/1

== system Project1_SPXMMA001/PLC Controller Suite/__Logic/Task/Program/__Logic/XIC16/Instruction_Enable/__CoreVarRead ==
  DataRead : DataStoreRead  DataStoreName=xxx_PLC_VAR_TL3_STOP  IndexOptions=Index vector (dialog)  Indices=1  OutputSizes=1
  y : Outport  VectorParamsAs1DForOutWhenUnconnected=off
  wires:
  DataRead/1 -> y/1

== system Project1_SPXMMA001/PLC Controller Suite/__Logic/Task/Program/__Logic/XIC16/RungInOverride/ForceRungInFalseRead ==
  __CoreLabelRead : Subsystem  Tag=CoreVarReadBlock  DisableCoverage=on  TreatAsAtomicUnit=on  mask{PLCBlockType=CoreLabelRead}
      mask init:
      | slplc.callbacks.initRoutineLabelRead(gcb);
      mask Help: web([docroot '/plccoder/ref/__corelabelread' '.html']);
      mask DialogControl PLCBlockTitle Prompt: Core Label Read
  Out1 : Outport  VectorParamsAs1DForOutWhenUnconnected=off
  wires:
  __CoreLabelRead/1(Out1) -> Out1/1

== system Project1_SPXMMA001/PLC Controller Suite/__Logic/Task/Program/__Logic/XIC2/BlockEnableRead/__CoreLabelRead ==
  DataRead : DataStoreRead  DataStoreName=x_PLCLabel__s4_3653__Block_Enable  IndexOptions=Index vector (dialog)  Indices=1  OutputSizes=1
  Out1 : Outport  VectorParamsAs1DForOutWhenUnconnected=off
  wires:
  DataRead/1 -> Out1/1

== system Project1_SPXMMA001/PLC Controller Suite/__Logic/Task/Program/__Logic/XIC2/Instruction_Enable/__CoreVarRead ==
  DataRead : DataStoreRead  DataStoreName=xxx_PLC_VAR_TOFF  DataStoreElements=xxx_PLC_VAR_TOFF.DN  IndexOptions=Index vector (dialog)  Indices=1  OutputSizes=1
  y : Outport  VectorParamsAs1DForOutWhenUnconnected=off
  wires:
  DataRead/1 -> y/1

== system Project1_SPXMMA001/PLC Controller Suite/__Logic/Task/Program/__Logic/XIC2/RungInOverride/ForceRungInFalseRead ==
  __CoreLabelRead : Subsystem  Tag=CoreVarReadBlock  DisableCoverage=on  TreatAsAtomicUnit=on  mask{PLCBlockType=CoreLabelRead}
      mask init:
      | slplc.callbacks.initRoutineLabelRead(gcb);
      mask Help: web([docroot '/plccoder/ref/__corelabelread' '.html']);
      mask DialogControl PLCBlockTitle Prompt: Core Label Read
  Out1 : Outport  VectorParamsAs1DForOutWhenUnconnected=off
  wires:
  __CoreLabelRead/1(Out1) -> Out1/1

== system Project1_SPXMMA001/PLC Controller Suite/__Logic/Task/Program/__Logic/XIC3/BlockEnableRead/__CoreLabelRead ==
  DataRead : DataStoreRead  DataStoreName=x_PLCLabel__s4_3653__Block_Enable  IndexOptions=Index vector (dialog)  Indices=1  OutputSizes=1
  Out1 : Outport  VectorParamsAs1DForOutWhenUnconnected=off
  wires:
  DataRead/1 -> Out1/1

== system Project1_SPXMMA001/PLC Controller Suite/__Logic/Task/Program/__Logic/XIC3/Instruction_Enable/__CoreVarRead ==
  DataRead : DataStoreRead  DataStoreName=xxx_PLC_VAR_TON  DataStoreElements=xxx_PLC_VAR_TON.DN  IndexOptions=Index vector (dialog)  Indices=1  OutputSizes=1
  y : Outport  VectorParamsAs1DForOutWhenUnconnected=off
  wires:
  DataRead/1 -> y/1

== system Project1_SPXMMA001/PLC Controller Suite/__Logic/Task/Program/__Logic/XIC3/RungInOverride/ForceRungInFalseRead ==
  __CoreLabelRead : Subsystem  Tag=CoreVarReadBlock  DisableCoverage=on  TreatAsAtomicUnit=on  mask{PLCBlockType=CoreLabelRead}
      mask init:
      | slplc.callbacks.initRoutineLabelRead(gcb);
      mask Help: web([docroot '/plccoder/ref/__corelabelread' '.html']);
      mask DialogControl PLCBlockTitle Prompt: Core Label Read
  Out1 : Outport  VectorParamsAs1DForOutWhenUnconnected=off
  wires:
  __CoreLabelRead/1(Out1) -> Out1/1

== system Project1_SPXMMA001/PLC Controller Suite/__Logic/Task/Program/__Logic/XIC4/BlockEnableRead/__CoreLabelRead ==
  DataRead : DataStoreRead  DataStoreName=x_PLCLabel__s4_3653__Block_Enable  IndexOptions=Index vector (dialog)  Indices=1  OutputSizes=1
  Out1 : Outport  VectorParamsAs1DForOutWhenUnconnected=off
  wires:
  DataRead/1 -> Out1/1

== system Project1_SPXMMA001/PLC Controller Suite/__Logic/Task/Program/__Logic/XIC4/Instruction_Enable/__CoreVarRead ==
  DataRead : DataStoreRead  DataStoreName=xxx_PLC_VAR_PED2_1  IndexOptions=Index vector (dialog)  Indices=1  OutputSizes=1
  y : Outport  VectorParamsAs1DForOutWhenUnconnected=off
  wires:
  DataRead/1 -> y/1

== system Project1_SPXMMA001/PLC Controller Suite/__Logic/Task/Program/__Logic/XIC4/RungInOverride/ForceRungInFalseRead ==
  __CoreLabelRead : Subsystem  Tag=CoreVarReadBlock  DisableCoverage=on  TreatAsAtomicUnit=on  mask{PLCBlockType=CoreLabelRead}
      mask init:
      | slplc.callbacks.initRoutineLabelRead(gcb);
      mask Help: web([docroot '/plccoder/ref/__corelabelread' '.html']);
      mask DialogControl PLCBlockTitle Prompt: Core Label Read
  Out1 : Outport  VectorParamsAs1DForOutWhenUnconnected=off
  wires:
  __CoreLabelRead/1(Out1) -> Out1/1

== system Project1_SPXMMA001/PLC Controller Suite/__Logic/Task/Program/__Logic/XIC5/BlockEnableRead/__CoreLabelRead ==
  DataRead : DataStoreRead  DataStoreName=x_PLCLabel__s4_3653__Block_Enable  IndexOptions=Index vector (dialog)  Indices=1  OutputSizes=1
  Out1 : Outport  VectorParamsAs1DForOutWhenUnconnected=off
  wires:
  DataRead/1 -> Out1/1

== system Project1_SPXMMA001/PLC Controller Suite/__Logic/Task/Program/__Logic/XIC5/Instruction_Enable/__CoreVarRead ==
  DataRead : DataStoreRead  DataStoreName=xxx_PLC_VAR_PED2_2  IndexOptions=Index vector (dialog)  Indices=1  OutputSizes=1
  y : Outport  VectorParamsAs1DForOutWhenUnconnected=off
  wires:
  DataRead/1 -> y/1

== system Project1_SPXMMA001/PLC Controller Suite/__Logic/Task/Program/__Logic/XIC5/RungInOverride/ForceRungInFalseRead ==
  __CoreLabelRead : Subsystem  Tag=CoreVarReadBlock  DisableCoverage=on  TreatAsAtomicUnit=on  mask{PLCBlockType=CoreLabelRead}
      mask init:
      | slplc.callbacks.initRoutineLabelRead(gcb);
      mask Help: web([docroot '/plccoder/ref/__corelabelread' '.html']);
      mask DialogControl PLCBlockTitle Prompt: Core Label Read
  Out1 : Outport  VectorParamsAs1DForOutWhenUnconnected=off
  wires:
  __CoreLabelRead/1(Out1) -> Out1/1

== system Project1_SPXMMA001/PLC Controller Suite/__Logic/Task/Program/__Logic/XIC6/BlockEnableRead/__CoreLabelRead ==
  DataRead : DataStoreRead  DataStoreName=x_PLCLabel__s4_3653__Block_Enable  IndexOptions=Index vector (dialog)  Indices=1  OutputSizes=1
  Out1 : Outport  VectorParamsAs1DForOutWhenUnconnected=off
  wires:
  DataRead/1 -> Out1/1

== system Project1_SPXMMA001/PLC Controller Suite/__Logic/Task/Program/__Logic/XIC6/Instruction_Enable/__CoreVarRead ==
  DataRead : DataStoreRead  DataStoreName=xxx_PLC_VAR_OFF  DataStoreElements=xxx_PLC_VAR_OFF.DN  IndexOptions=Index vector (dialog)  Indices=1  OutputSizes=1
  y : Outport  VectorParamsAs1DForOutWhenUnconnected=off
  wires:
  DataRead/1 -> y/1

== system Project1_SPXMMA001/PLC Controller Suite/__Logic/Task/Program/__Logic/XIC6/RungInOverride/ForceRungInFalseRead ==
  __CoreLabelRead : Subsystem  Tag=CoreVarReadBlock  DisableCoverage=on  TreatAsAtomicUnit=on  mask{PLCBlockType=CoreLabelRead}
      mask init:
      | slplc.callbacks.initRoutineLabelRead(gcb);
      mask Help: web([docroot '/plccoder/ref/__corelabelread' '.html']);
      mask DialogControl PLCBlockTitle Prompt: Core Label Read
  Out1 : Outport  VectorParamsAs1DForOutWhenUnconnected=off
  wires:
  __CoreLabelRead/1(Out1) -> Out1/1

== system Project1_SPXMMA001/PLC Controller Suite/__Logic/Task/Program/__Logic/XIC7/BlockEnableRead/__CoreLabelRead ==
  DataRead : DataStoreRead  DataStoreName=x_PLCLabel__s4_3653__Block_Enable  IndexOptions=Index vector (dialog)  Indices=1  OutputSizes=1
  Out1 : Outport  VectorParamsAs1DForOutWhenUnconnected=off
  wires:
  DataRead/1 -> Out1/1

== system Project1_SPXMMA001/PLC Controller Suite/__Logic/Task/Program/__Logic/XIC7/Instruction_Enable/__CoreVarRead ==
  DataRead : DataStoreRead  DataStoreName=xxx_PLC_VAR_ON  DataStoreElements=xxx_PLC_VAR_ON.DN  IndexOptions=Index vector (dialog)  Indices=1  OutputSizes=1
  y : Outport  VectorParamsAs1DForOutWhenUnconnected=off
  wires:
  DataRead/1 -> y/1

== system Project1_SPXMMA001/PLC Controller Suite/__Logic/Task/Program/__Logic/XIC7/RungInOverride/ForceRungInFalseRead ==
  __CoreLabelRead : Subsystem  Tag=CoreVarReadBlock  DisableCoverage=on  TreatAsAtomicUnit=on  mask{PLCBlockType=CoreLabelRead}
      mask init:
      | slplc.callbacks.initRoutineLabelRead(gcb);
      mask Help: web([docroot '/plccoder/ref/__corelabelread' '.html']);
      mask DialogControl PLCBlockTitle Prompt: Core Label Read
  Out1 : Outport  VectorParamsAs1DForOutWhenUnconnected=off
  wires:
  __CoreLabelRead/1(Out1) -> Out1/1

== system Project1_SPXMMA001/PLC Controller Suite/__Logic/Task/Program/__Logic/XIC8/BlockEnableRead/__CoreLabelRead ==
  DataRead : DataStoreRead  DataStoreName=x_PLCLabel__s4_3653__Block_Enable  IndexOptions=Index vector (dialog)  Indices=1  OutputSizes=1
  Out1 : Outport  VectorParamsAs1DForOutWhenUnconnected=off
  wires:
  DataRead/1 -> Out1/1

== system Project1_SPXMMA001/PLC Controller Suite/__Logic/Task/Program/__Logic/XIC8/Instruction_Enable/__CoreVarRead ==
  DataRead : DataStoreRead  DataStoreName=xxx_PLC_VAR_ZONE1  IndexOptions=Index vector (dialog)  Indices=1  OutputSizes=1
  y : Outport  VectorParamsAs1DForOutWhenUnconnected=off
  wires:
  DataRead/1 -> y/1

== system Project1_SPXMMA001/PLC Controller Suite/__Logic/Task/Program/__Logic/XIC8/RungInOverride/ForceRungInFalseRead ==
  __CoreLabelRead : Subsystem  Tag=CoreVarReadBlock  DisableCoverage=on  TreatAsAtomicUnit=on  mask{PLCBlockType=CoreLabelRead}
      mask init:
      | slplc.callbacks.initRoutineLabelRead(gcb);
      mask Help: web([docroot '/plccoder/ref/__corelabelread' '.html']);
      mask DialogControl PLCBlockTitle Prompt: Core Label Read
  Out1 : Outport  VectorParamsAs1DForOutWhenUnconnected=off
  wires:
  __CoreLabelRead/1(Out1) -> Out1/1

== system Project1_SPXMMA001/PLC Controller Suite/__Logic/Task/Program/__Logic/XIC9/BlockEnableRead/__CoreLabelRead ==
  DataRead : DataStoreRead  DataStoreName=x_PLCLabel__s4_3653__Block_Enable  IndexOptions=Index vector (dialog)  Indices=1  OutputSizes=1
  Out1 : Outport  VectorParamsAs1DForOutWhenUnconnected=off
  wires:
  DataRead/1 -> Out1/1

== system Project1_SPXMMA001/PLC Controller Suite/__Logic/Task/Program/__Logic/XIC9/Instruction_Enable/__CoreVarRead ==
  DataRead : DataStoreRead  DataStoreName=xxx_PLC_VAR_T2OFF  DataStoreElements=xxx_PLC_VAR_T2OFF.DN  IndexOptions=Index vector (dialog)  Indices=1  OutputSizes=1
  y : Outport  VectorParamsAs1DForOutWhenUnconnected=off
  wires:
  DataRead/1 -> y/1

== system Project1_SPXMMA001/PLC Controller Suite/__Logic/Task/Program/__Logic/XIC9/RungInOverride/ForceRungInFalseRead ==
  __CoreLabelRead : Subsystem  Tag=CoreVarReadBlock  DisableCoverage=on  TreatAsAtomicUnit=on  mask{PLCBlockType=CoreLabelRead}
      mask init:
      | slplc.callbacks.initRoutineLabelRead(gcb);
      mask Help: web([docroot '/plccoder/ref/__corelabelread' '.html']);
      mask DialogControl PLCBlockTitle Prompt: Core Label Read
  Out1 : Outport  VectorParamsAs1DForOutWhenUnconnected=off
  wires:
  __CoreLabelRead/1(Out1) -> Out1/1

== system Project1_SPXMMA001/PLC Controller Suite/__Logic/Task/Program/__Logic/XIO1/BlockEnableRead/__CoreLabelRead ==
  DataRead : DataStoreRead  DataStoreName=x_PLCLabel__s4_3653__Block_Enable  IndexOptions=Index vector (dialog)  Indices=1  OutputSizes=1
  Out1 : Outport  VectorParamsAs1DForOutWhenUnconnected=off
  wires:
  DataRead/1 -> Out1/1

== system Project1_SPXMMA001/PLC Controller Suite/__Logic/Task/Program/__Logic/XIO1/Instruction_Enable/__CoreVarRead ==
  DataRead : DataStoreRead  DataStoreName=xxx_PLC_VAR_ZONE2_SENSOR  IndexOptions=Index vector (dialog)  Indices=1  OutputSizes=1
  y : Outport  VectorParamsAs1DForOutWhenUnconnected=off
  wires:
  DataRead/1 -> y/1
